simulink model "tema"  (R2017a)
settings: Solver=VariableStepAuto  StartTime=0.0  StopTime=10.0  RelTol=1e-3
values from neighbouring files (symbols this model uses):
  a1 = 1.31 / 10^4    (= 0.000131)    [load_workspace_a.m]    (also in load_workspace_b.m; load_workspace_c.m; load_workspace_d.m; load_workspace_e.m)
  A1 = 0.06    [load_workspace_a.m]    (also in load_workspace_b.m; load_workspace_c.m; load_workspace_d.m; load_workspace_e.m)
  a2 = 1.51 / 10^4    (= 0.000151)    [load_workspace_a.m]    (also in load_workspace_b.m; load_workspace_c.m; load_workspace_d.m; load_workspace_e.m)
  A2 = 0.06    [load_workspace_a.m]    (also in load_workspace_b.m; load_workspace_c.m; load_workspace_d.m; load_workspace_e.m)
  A3 = 0.06    [load_workspace_a.m]    (also in load_workspace_b.m; load_workspace_c.m; load_workspace_d.m; load_workspace_e.m)
  a3 = 9.27 / 10^5    (= 9.27e-05)    [load_workspace_a.m]    (also in load_workspace_b.m; load_workspace_c.m; load_workspace_d.m; load_workspace_e.m)
  a4 = 8.82 / 10^5    (= 8.82e-05)    [load_workspace_a.m]    (also in load_workspace_b.m; load_workspace_c.m; load_workspace_d.m; load_workspace_e.m)
  A4 = 0.06    [load_workspace_a.m]    (also in load_workspace_b.m; load_workspace_c.m; load_workspace_d.m; load_workspace_e.m)
  ac = 4.307 / 10^6    (= 4.307e-06)    [load_workspace_a.m]    (also in load_workspace_b.m; load_workspace_c.m; load_workspace_d.m; load_workspace_e.m)
  AT = 0.1273    [load_workspace_a.m]    (also in load_workspace_b.m; load_workspace_c.m; load_workspace_d.m; load_workspace_e.m)
  g = 9.8    [load_workspace_a.m]    (also in load_workspace_b.m; load_workspace_c.m; load_workspace_d.m; load_workspace_e.m)
  kp = 0.5 / 10^4    (= 5e-05)    [load_workspace_a.m]    (also in load_workspace_b.m; load_workspace_c.m; load_workspace_d.m; load_workspace_e.m)
  l1 = 2/4    (= 0.5)    [load_workspace_a.m]    (also in load_workspace_b.m; load_workspace_c.m; load_workspace_d.m; load_workspace_e.m)
  l2 = 3/4    (= 0.75)    [load_workspace_a.m]    (also in load_workspace_b.m; load_workspace_c.m; load_workspace_d.m; load_workspace_e.m)
  q = 1000    [load_workspace_a.m]    (also in load_workspace_b.m; load_workspace_c.m; load_workspace_d.m; load_workspace_e.m)
settings Model: Creator=pangi  LastModifiedBy=pangi

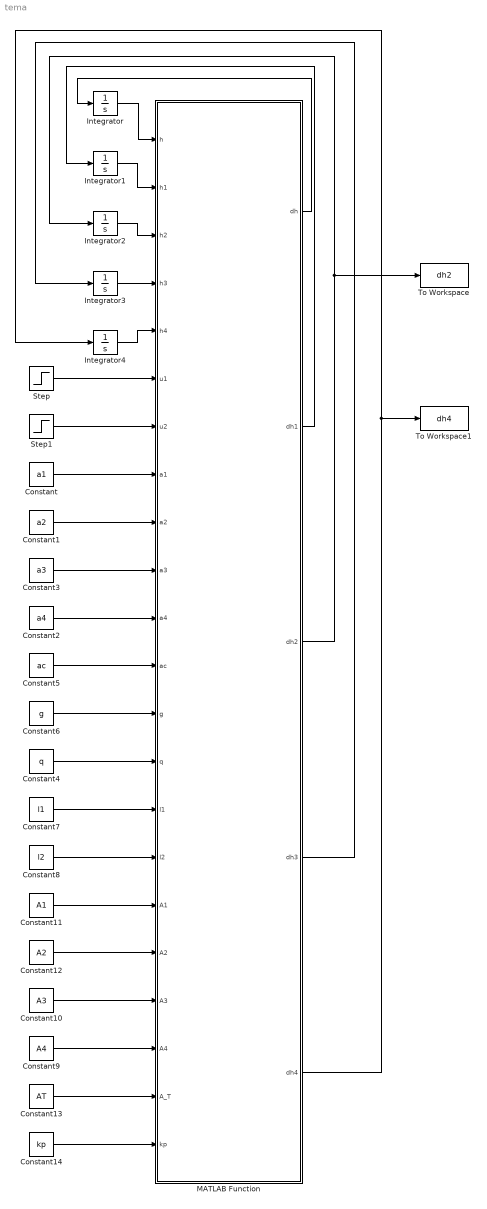
== system tema ==
  Constant : Constant  Value=a1
  Constant1 : Constant  Value=a2
  Constant10 : Constant  Value=A3
  Constant11 : Constant  Value=A1
  Constant12 : Constant  Value=A2
  Constant13 : Constant  Value=AT
  Constant14 : Constant  Value=kp
  Constant2 : Constant  Value=a4
  Constant3 : Constant  Value=a3
  Constant4 : Constant  Value=q
  Constant5 : Constant  Value=ac
  Constant6 : Constant  Value=g
  Constant7 : Constant  Value=l1
  Constant8 : Constant  Value=l2
  Constant9 : Constant  Value=A4
  Integrator{,1..4} (5 alike) : Integrator
  MATLAB Function : MATLAB Function  TreatAsAtomicUnit=on
  Step : Step  SampleTime=0
  Step1 : Step  SampleTime=0
  To Workspace : ToWorkspace  VariableName=dh2  SaveFormat=Timeseries  SampleTime=-1
  To Workspace1 : ToWorkspace  VariableName=dh4  SaveFormat=Timeseries  SampleTime=-1
  wires:
  MATLAB Function/1(dh) -> Integrator/1
  MATLAB Function/2(dh1) -> Integrator1/1
  MATLAB Function/3(dh2) -> To Workspace/1, Integrator2/1
  MATLAB Function/4(dh3) -> Integrator3/1
  MATLAB Function/5(dh4) -> To Workspace1/1, Integrator4/1
  Integrator/1 -> MATLAB Function/1(h)
  Integrator1/1 -> MATLAB Function/2(h1)
  Integrator2/1 -> MATLAB Function/3(h2)
  Integrator3/1 -> MATLAB Function/4(h3)
  Integrator4/1 -> MATLAB Function/5(h4)
  Step/1 -> MATLAB Function/6(u1)
  Step1/1 -> MATLAB Function/7(u2)
  Constant/1 -> MATLAB Function/8(a1)
  Constant1/1 -> MATLAB Function/9(a2)
  Constant3/1 -> MATLAB Function/10(a3)
  Constant2/1 -> MATLAB Function/11(a4)
  Constant5/1 -> MATLAB Function/12(ac)
  Constant6/1 -> MATLAB Function/13(g)
  Constant4/1 -> MATLAB Function/14(q)
  Constant7/1 -> MATLAB Function/15(l1)
  Constant8/1 -> MATLAB Function/16(l2)
  Constant11/1 -> MATLAB Function/17(A1)
  Constant12/1 -> MATLAB Function/18(A2)
  Constant10/1 -> MATLAB Function/19(A3)
  Constant9/1 -> MATLAB Function/20(A4)
  Constant13/1 -> MATLAB Function/21(A_T)
  Constant14/1 -> MATLAB Function/22(kp)

== matlab function tema/MATLAB Function ==
  data: dh output; h input; h1 input; h2 input; h3 input; h4 input; u1 input; dh1 output; dh2 output; dh3 output; dh4 output; u2 input; a1 input; a2 input; a3 input; a4 input; ac input; g input; q input; l1 input; l2 input; A1 input; A2 input; A3 input; A4 input; A_T input; kp input
function [dh, dh1, dh2, dh3, dh4] = fcn(h, h1, h2, h3, h4, u1, u2, a1, a2, a3, a4, ac, g, q, l1, l2, A1, A2, A3, A4, A_T, kp)
    dh1 = 1/A1*(-a1*sqrt(2*g*h1) - ac*sign(q*g*h1 - q*g*h2)*sqrt(2*g*abs(h1 - h2)) + a3*sqrt(2*g*h3) + l1*kp*u1);
    dh2 = 1/A2*(-a2*sqrt(2*g*h2) - ac*sign(q*g*h1 - q*g*h2)*sqrt(2*g*abs(h1 - h2)) + a4*sqrt(2*g*h4) + l2*kp*u2);
    dh3 = 1/A3*(-a3*sqrt(2*g*h3) + (1 - l2)*kp*u2);
    dh4 = 1/A4*(-a4*sqrt(2*g*h4) + (1 - l1)*kp*u1);
    dh = 1/AT*(a1*sqrt(2*g*h1) + a2*sqrt(2*g*h2) - kp*u1 - kp*u2);
end
